simulink model "IMcontrol0"  (Simulink 10.0)
settings: Solver=ode23tb  StartTime=0.0  StopTime=1  MaxStep=1e-4  RelTol=1e-3
undefined symbols (not defined in the file): DiscIntNeverNeededParam
libraries: powerlib x4, simulink x1
settings Model: Creator=80573  LastModifiedBy=Inspiron
settings DataIOCC: SaveFormat=Dataset
settings OptimizationCC: LifeSpan=auto
settings DebuggingCC: UnderspecifiedInitializationDetection=Simplified  MergeDetectMultiDrivingBlocksExec=error  SFUnexpectedBacktrackingDiag=error  SFNoUnconditionalDefaultTransitionDiag=error  SFExecutionAtInitializationDiag=warning
settings HardwareCC: ProdBitPerPointer=64  ProdBitPerSizeT=64  ProdBitPerPtrDiffT=64  ProdLargestAtomicFloat=Float  ProdIntDivRoundTo=Zero  ProdEndianess=LittleEndian  ProdWordSize=64  ProdHWDeviceType=Intel->x86-64 (Windows64)
settings ModelReferenceCC: PropagateSignalLabelsOutOfModel=on
settings CodeAppCC: StateflowObjectComments=off
settings GRTTargetCC: TargetLangStandard=C99 (ISO)  CombineOutputUpdateFcns=on  GRTInterface=off
settings ConfigComp: CovMetricSettings=dwe  CovHtmlReporting=off  CovSaveCumulativeToWorkspaceVar=off  CovSaveSingleToWorkspaceVar=off

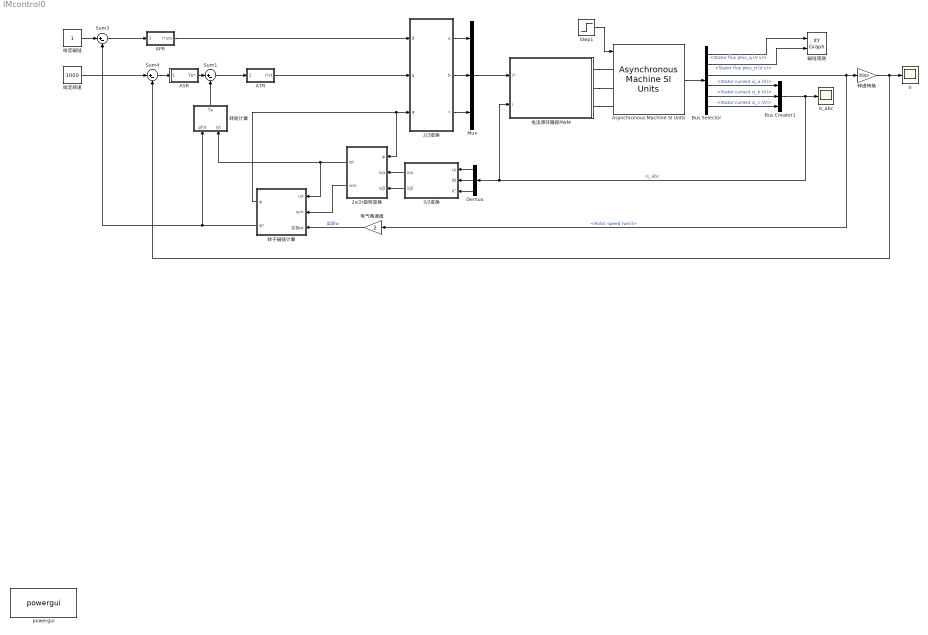
== system IMcontrol0 ==
  2/3变换 : Subsystem
  2s/2r旋转变换 : Subsystem
  3/2变换 : Subsystem
  AFR : Subsystem
  ASR : Subsystem
  ATR : Subsystem
  Asynchronous Machine SI Units : powerlib/Machines/Asynchronous Machine SI Units  RotorType=Squirrel-cage  PresetModel=No  MechanicalLoad=Torque Tm  ShowDetailedParameters=on  ReferenceFrame=Stationary  Units=SI  MeasurementBus=off  NominalParameters=[2200 380 50]  Stator=[0.435 0.002]  Rotor=[0.816 0.002]  Cage1=[0.4155 0.002066]  Cage2=[0.4168 0.0003495]  Lm=0.069  Mechanical=[0.19 0 2]  PolePairs=2  InitialConditions=[1 0 0 0 0 0 0 0]  SimulateSaturation=off  Saturation=[14.03593122, 27.81365428, 53.79336849, 72.68890987, 97.98006896, 148.6815601, 215.7428561, 302.9841135, 428.7778367 ; 230, 322, 414, 460, 506, 552, 598, 644, 690]  LoadFlowParameters=1492000  TsPowergui=0  TsBlock=-1  IterativeModel=Trapezoidal non iterative  IterativeDiscreteModel=Trapezoidal non iterative  Pmec=1.492e+006
      settings: SourceProductName=Simscape Electrical
  Bus Creator1 : BusCreator  Inputs=3
  Bus Selector : BusSelector  OutputSignals=Stator measurements.Stator flux phis_q (V s),Stator measurements.Stator flux phis_d (V s),Mechanical.Rotor speed (wm),Stator measurements.Stator current is_a (A),Stator measurements.Stator current is_b (A),Stator measurements.Stator current is_c (A)
  Demux : Demux  Outputs=3
  Mux : Mux  Inputs=3
  Step1 : Step  Time=0.6  After=55  SampleTime=0
  Sum1 : Sum  Inputs=|+-
  Sum3 : Sum  Inputs=|+-
  Sum4 : Sum  Inputs=|+-
  is_abc : Scope
  n : Scope
  powergui : powerlib/powergui  SimulationMode=Discrete  SampleTime=0.00001  frequency=50  Iterations=50  frequencyindice=50  Pbase=100e6  ErrMax=1e-4  UnitsV=kV  UnitsW=MW  buscounter=0  FunctionMessages=off  echomessages=off  EnableUseOfTLC=off  CurrentSourceSwitches=off  DisableSnubberDevices=off  DisableRonSwitches=off  DisableVfSwitches=off  DisplayEquations=off  AutomaticDiscreteSolvers=off  SolverType=Tustin/Backward Euler (TBE)  Interpol=off  ExternalGateDelay=off  methode=off  Ts=100  x0status=zero  SPID=on  SwTol=0  HookPort=off  NonlinearTolerance=1e-4  nMaxIteration=100  ContinueOnMaxIteration=off  RestoreLinks=warning  ResistiveCurrentMeasurement=off  Frange=[0:2:500]  Ylog=off  Xlog=on  ShowGrid=off  save=off  variable=ZData  structure=0  ZoomFFT=on  StartTime=0.0  cycles=1  DisplayStyle=1  fundamental=60  FreqAxis=off  MaxFrequency=1000  frequencyindicesteady=1  RmsSteady=1  display=off
      settings: SourceProductName=Simscape Electrical
  电气角速度 : Gain  Gain=2
  电流滞环跟踪PWM : Subsystem
  磁链观测 : simulink/Sinks/XY Graph  xmin=-1  xmax=1  ymin=-1  ymax=1  st=-1
  给定磁链 : Constant
  给定转速 : Constant  Value=1000
  转子磁链计算 : Subsystem
  转矩计算 : MATLAB Function  TreatAsAtomicUnit=on
  转速转换 : Gain  Gain=30/pi
  wires:
  Step1/1 -> Asynchronous Machine SI Units/1
  Sum1/1 -> ATR/1(" ")
  Sum3/1 -> AFR/1(" ")
  Sum4/1 -> ASR/1("  ")
  给定磁链/1 -> Sum3/1
  ATR/1(i*st) -> 2/3变换/2(q)
  2/3变换/2(b) -> Mux/2
  2/3变换/3(c) -> Mux/3
  AFR/1(i*sm) -> 2/3变换/1(d)
  2/3变换/1(a) -> Mux/1
  Bus Selector/4 -> Bus Creator1/1  "<Stator current is_a (A)>"
  Bus Selector/6 -> Bus Creator1/3  "<Stator current is_c (A)>"
  Bus Selector/1 -> 磁链观测/1  "<Stator flux phis_q (V s)>"
  Bus Selector/2 -> 磁链观测/2  "<Stator flux phis_d (V s)>"
  Bus Selector/5 -> Bus Creator1/2  "<Stator current is_b (A)>"
  Bus Selector/3 -> 电气角速度/1, 转速转换/1  "<Rotor speed (wm)>"
  Bus Creator1/1 -> 电流滞环跟踪PWM/2(i), Demux/1, is_abc/1  "is_abc"
  Asynchronous Machine SI Units/1 -> Bus Selector/1
  Mux/1 -> 电流滞环跟踪PWM/1(i*)
  ASR/1(Te*) -> Sum1/1
  转矩计算/1(Te) -> Sum1/2
  Demux/1 -> 3/2变换/1(iA)
  Demux/2 -> 3/2变换/2(iB)
  Demux/3 -> 3/2变换/3(iC)
  2s/2r旋转变换/1(ist) -> 转矩计算/2(ist), 转子磁链计算/1(ist)
  3/2变换/1(isα) -> 2s/2r旋转变换/2(isα)
  3/2变换/2(isβ) -> 2s/2r旋转变换/3(isβ)
  给定转速/1 -> Sum4/1
  转速转换/1 -> Sum4/2, n/1
  转子磁链计算/2(ψr) -> Sum3/2, 转矩计算/1(phir)
  转子磁链计算/1(φ) -> 2s/2r旋转变换/1(φ), 2/3变换/3(φ)
  电气角速度/1 -> 转子磁链计算/3(实际w)  "实际w"
  2s/2r旋转变换/2(ism) -> 转子磁链计算/2(ism)
  connections:
  电流滞环跟踪PWM/RConn1 -- Asynchronous Machine SI Units/LConn1
  电流滞环跟踪PWM/RConn2 -- Asynchronous Machine SI Units/LConn2
  电流滞环跟踪PWM/RConn3 -- Asynchronous Machine SI Units/LConn3

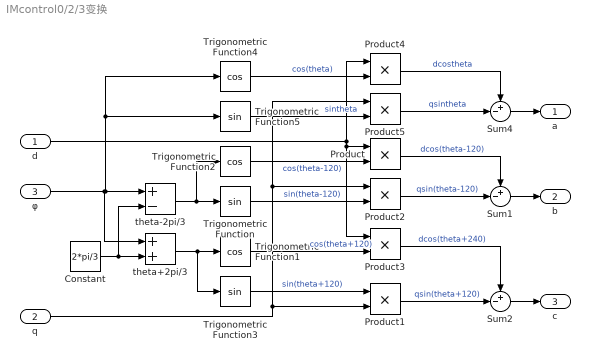
== system IMcontrol0/2/3变换 ==
  d : Inport
  q : Inport  Port=2
  φ : Inport  Port=3
  Constant : Constant  Value=2*pi/3
  Product{,1..5} (6 alike) : Product
  Sum1 : Sum  Inputs=+-|
  Sum2 : Sum  Inputs=+-|
  Sum4 : Sum  Inputs=+-|
  Trigonometric Function : Trigonometry
  Trigonometric Function1 : Trigonometry  Operator=cos
  Trigonometric Function2 : Trigonometry  Operator=cos
  Trigonometric Function3 : Trigonometry
  Trigonometric Function4 : Trigonometry  Operator=cos
  Trigonometric Function5 : Trigonometry
  theta+2pi/3 : Sum
  theta-2pi/3 : Sum  Inputs=+-
  a : Outport  VectorParamsAs1DForOutWhenUnconnected=off
  b : Outport  Port=2  VectorParamsAs1DForOutWhenUnconnected=off
  c : Outport  Port=3  VectorParamsAs1DForOutWhenUnconnected=off
  wires:
  Trigonometric Function5/1 -> Product5/2  "sintheta"
  Product/1 -> Sum1/1  "dcos(theta-120)"
  Trigonometric Function1/1 -> Product3/2  "cos(theta+120)"
  Product3/1 -> Sum2/1  "dcos(theta+240)"
  d/1 -> Product/1, Product3/1, Product4/1
  Constant/1 -> theta+2pi/3/2, theta-2pi/3/2
  φ/1 -> Trigonometric Function4/1, Trigonometric Function5/1, theta-2pi/3/1, theta+2pi/3/1
  theta+2pi/3/1 -> Trigonometric Function3/1, Trigonometric Function1/1
  q/1 -> Product5/1, Product2/1, Product1/2
  Trigonometric Function/1 -> Product2/2  "sin(theta-120)"
  Product4/1 -> Sum4/1  "dcostheta"
  Product5/1 -> Sum4/2  "qsintheta"
  theta-2pi/3/1 -> Trigonometric Function2/1, Trigonometric Function/1
  Product1/1 -> Sum2/2  "qsin(theta+120)"
  Trigonometric Function2/1 -> Product/2  "cos(theta-120)"
  Sum4/1 -> a/1
  Sum1/1 -> b/1
  Trigonometric Function4/1 -> Product4/2  "cos(theta)"
  Trigonometric Function3/1 -> Product1/1  "sin(theta+120)"
  Product2/1 -> Sum1/2  "qsin(theta-120)"
  Sum2/1 -> c/1

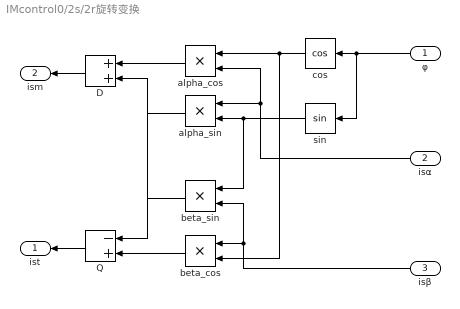
== system IMcontrol0/2s/2r旋转变换 ==
  φ : Inport
  isα : Inport  Port=2
  isβ : Inport  Port=3
  D : Sum
  Q : Sum  Inputs=-+
  alpha_cos : Product
  alpha_sin : Product
  beta_cos : Product
  beta_sin : Product
  cos : Trigonometry  Operator=cos
  sin : Trigonometry
  ist : Outport
  ism : Outport  Port=2
  wires:
  cos/1 -> beta_cos/2, alpha_cos/1
  beta_cos/1 -> Q/2
  sin/1 -> beta_sin/1, alpha_sin/2
  isα/1 -> alpha_cos/2, alpha_sin/1
  alpha_sin/1 -> Q/1
  beta_sin/1 -> D/2
  isβ/1 -> beta_sin/2, beta_cos/1
  φ/1 -> sin/1, cos/1
  D/1 -> ism/1
  alpha_cos/1 -> D/1
  Q/1 -> ist/1

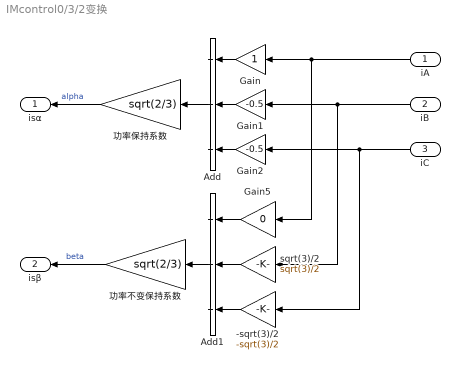
== system IMcontrol0/3/2变换 ==
  iA : Inport
  iB : Inport  Port=2
  iC : Inport  Port=3
  -sqrt(3)/2 : Gain  Gain=-sqrt(3)/2
  Add : Sum  Inputs=3
  Add1 : Sum  Inputs=3
  Gain : Gain
  Gain1 : Gain  Gain=-0.5
  Gain2 : Gain  Gain=-0.5
  Gain5 : Gain  Gain=0
  sqrt(3)/2 : Gain  Gain=sqrt(3)/2
  功率不变保持系数 : Gain  Gain=sqrt(2/3)
  功率保持系数 : Gain  Gain=sqrt(2/3)
  isα : Outport
  isβ : Outport  Port=2
  wires:
  sqrt(3)/2/1 -> Add1/2
  Gain/1 -> Add/1
  -sqrt(3)/2/1 -> Add1/3
  iB/1 -> sqrt(3)/2/1, Gain1/1
  Add/1 -> 功率保持系数/1
  Gain1/1 -> Add/2
  Gain5/1 -> Add1/1
  iA/1 -> Gain5/1, Gain/1
  Gain2/1 -> Add/3
  iC/1 -> -sqrt(3)/2/1, Gain2/1
  Add1/1 -> 功率不变保持系数/1
  功率不变保持系数/1 -> isβ/1  "beta"
  功率保持系数/1 -> isα/1  "alpha"

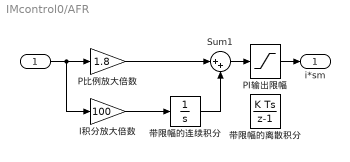
== system IMcontrol0/AFR ==
  " " : Inport
  I积分放大倍数 : Gain  Gain=100
  PI输出限幅 : Saturate  UpperLimit=13  LowerLimit=-13
  P比例放大倍数 : Gain  Gain=1.8
  Sum1 : Sum  Inputs=|++
  带限幅的离散积分 : DiscreteIntegrator  SampleTime=2e-5  ICPrevOutput=DiscIntNeverNeededParam  ICPrevScaledInput=DiscIntNeverNeededParam
  带限幅的连续积分 : Integrator  LimitOutput=on  UpperSaturationLimit=15  LowerSaturationLimit=-15
  i*sm : Outport  VectorParamsAs1DForOutWhenUnconnected=off
  wires:
  Sum1/1 -> PI输出限幅/1
  PI输出限幅/1 -> i*sm/1
  I积分放大倍数/1 -> 带限幅的连续积分/1
  P比例放大倍数/1 -> Sum1/1
  带限幅的连续积分/1 -> Sum1/2
  " "/1 -> I积分放大倍数/1, P比例放大倍数/1

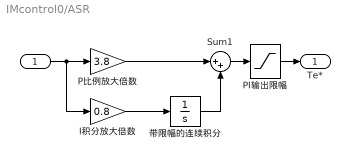
== system IMcontrol0/ASR ==
  "  " : Inport
  I积分放大倍数 : Gain  Gain=0.8
  PI输出限幅 : Saturate  UpperLimit=75  LowerLimit=-75
  P比例放大倍数 : Gain  Gain=3.8
  Sum1 : Sum  Inputs=|++
  带限幅的连续积分 : Integrator  LimitOutput=on  UpperSaturationLimit=80  LowerSaturationLimit=-80
  Te* : Outport  VectorParamsAs1DForOutWhenUnconnected=off
  wires:
  Sum1/1 -> PI输出限幅/1
  PI输出限幅/1 -> Te*/1
  P比例放大倍数/1 -> Sum1/1
  I积分放大倍数/1 -> 带限幅的连续积分/1
  带限幅的连续积分/1 -> Sum1/2
  "  "/1 -> I积分放大倍数/1, P比例放大倍数/1

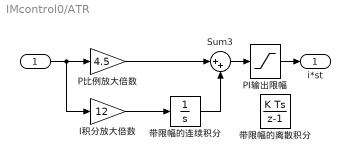
== system IMcontrol0/ATR ==
  " " : Inport
  I积分放大倍数 : Gain  Gain=12
  PI输出限幅 : Saturate  UpperLimit=60  LowerLimit=-60
  P比例放大倍数 : Gain  Gain=4.5
  Sum3 : Sum  Inputs=|++
  带限幅的离散积分 : DiscreteIntegrator  SampleTime=2e-5  ICPrevOutput=DiscIntNeverNeededParam  ICPrevScaledInput=DiscIntNeverNeededParam
  带限幅的连续积分 : Integrator  LimitOutput=on  UpperSaturationLimit=65  LowerSaturationLimit=-65
  i*st : Outport  VectorParamsAs1DForOutWhenUnconnected=off
  wires:
  Sum3/1 -> PI输出限幅/1
  P比例放大倍数/1 -> Sum3/1
  " "/1 -> I积分放大倍数/1, P比例放大倍数/1
  PI输出限幅/1 -> i*st/1
  带限幅的连续积分/1 -> Sum3/2
  I积分放大倍数/1 -> 带限幅的连续积分/1

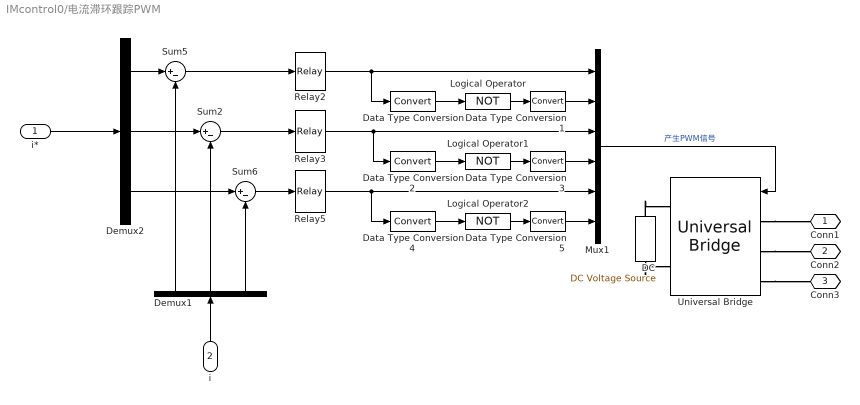
== system IMcontrol0/电流滞环跟踪PWM ==
  i* : Inport
  i : Inport  Port=2
  DC : powerlib/Electrical Sources/DC Voltage Source  Amplitude=510  Measurements=None
      settings: SourceProductName=Simscape Electrical
  Data Type Conversion{,1..5} (6 alike) : DataTypeConversion
  Demux1 : Demux  Outputs=3
  Demux2 : Demux  Outputs=3
  Logical Operator : Logic  Operator=NOT  Inputs=1  AllPortsSameDT=off
  Logical Operator1 : Logic  Operator=NOT  Inputs=1  AllPortsSameDT=off
  Logical Operator2 : Logic  Operator=NOT  Inputs=1  AllPortsSameDT=off
  Mux1 : Mux  Inputs=6
  Relay2 : Relay  OnSwitchValue=0.2  OffSwitchValue=-0.2  ZeroCross=off
  Relay3 : Relay  OnSwitchValue=0.2  OffSwitchValue=-0.2  ZeroCross=off
  Relay5 : Relay  OnSwitchValue=0.2  OffSwitchValue=-0.2  ZeroCross=off
  Sum2 : Sum  Inputs=|+-
  Sum5 : Sum  Inputs=|+-
  Sum6 : Sum  Inputs=|+-
  Universal Bridge : powerlib/Power Electronics/Universal Bridge  Arms=3  SnubberResistance=1e5  SnubberCapacitance=inf  Device=IGBT / Diodes  Ron=1e-3  Lon=0  ForwardVoltages="[  0  0  ]"  ForwardVoltage=0  GTOparameters=[ 10e-6 , 20e-6 ]  IGBTparameters=[ 1e-6 , 2e-6 ]  Measurements=None  Measurements_2=None  converterType=Rectifier
      settings: SourceProductName=Simscape Electrical
  Conn1 : PMIOPort  Side=Right
  Conn2 : PMIOPort  Port=2  Side=Right
  Conn3 : PMIOPort  Port=3  Side=Right
  wires:
  Sum6/1 -> Relay5/1
  Data Type Conversion1/1 -> Mux1/2
  Sum5/1 -> Relay2/1
  Relay5/1 -> Data Type Conversion4/1, Mux1/5
  Data Type Conversion3/1 -> Mux1/4
  Relay2/1 -> Data Type Conversion/1, Mux1/1
  Relay3/1 -> Data Type Conversion2/1, Mux1/3
  Mux1/1 -> Universal Bridge/1  "产生PWM信号"
  Demux1/3 -> Sum6/2
  i/1 -> Demux1/1
  Demux2/1 -> Sum5/1
  Logical Operator2/1 -> Data Type Conversion5/1
  Data Type Conversion/1 -> Logical Operator/1
  i*/1 -> Demux2/1
  Logical Operator/1 -> Data Type Conversion1/1
  Demux1/2 -> Sum2/2
  Data Type Conversion5/1 -> Mux1/6
  Data Type Conversion2/1 -> Logical Operator1/1
  Demux1/1 -> Sum5/2
  Demux2/3 -> Sum6/1
  Demux2/2 -> Sum2/1
  Data Type Conversion4/1 -> Logical Operator2/1
  Sum2/1 -> Relay3/1
  Logical Operator1/1 -> Data Type Conversion3/1
  connections:
  DC/LConn1 -- Universal Bridge/RConn2
  DC/RConn1 -- Universal Bridge/RConn1
  Universal Bridge/LConn1 -- Conn1/RConn1
  Universal Bridge/LConn2 -- Conn2/RConn1
  Universal Bridge/LConn3 -- Conn3/RConn1

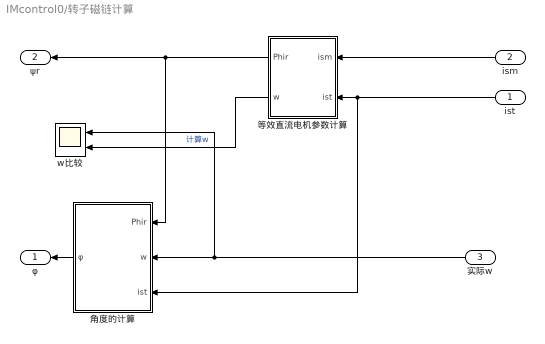
== system IMcontrol0/转子磁链计算 ==
  ist : Inport
  ism : Inport  Port=2
  实际w : Inport  Port=3
  w比较 : Scope  NumInputPorts=2
  等效直流电机参数计算 : Subsystem
  角度的计算 : Subsystem
  φ : Outport
  ψr : Outport  Port=2
  wires:
  等效直流电机参数计算/1(Phir) -> ψr/1, 角度的计算/1(Phir)
  实际w/1 -> w比较/1, 角度的计算/2(w)
  ist/1 -> 角度的计算/3(ist), 等效直流电机参数计算/2(ist)
  等效直流电机参数计算/2(w) -> w比较/2  "计算w"
  角度的计算/1(φ) -> φ/1
  ism/1 -> 等效直流电机参数计算/1(ism)

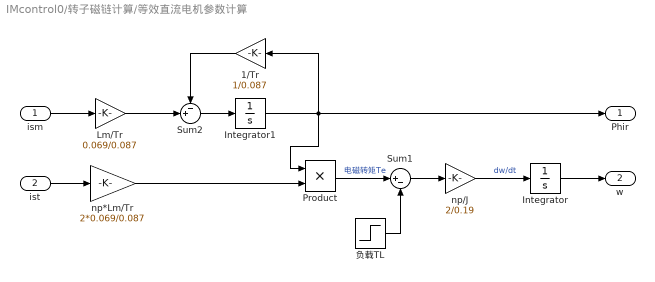
== system IMcontrol0/转子磁链计算/等效直流电机参数计算 ==
  ism : Inport
  ist : Inport  Port=2
  1/Tr : Gain  Gain=1/0.087
  Integrator : Integrator
  Integrator1 : Integrator  InitialCondition=1e-5
  Lm/Tr : Gain  Gain=0.069/0.087
  Product : Product
  Sum1 : Sum  Inputs=|+-
  Sum2 : Sum  Inputs=-+|
  np*Lm/Tr : Gain  Gain=2*0.069/0.087
  np/J : Gain  Gain=2/0.19
  负载TL : Step  Time=0.6  After=55  SampleTime=0
  Phir : Outport  VectorParamsAs1DForOutWhenUnconnected=off
  w : Outport  Port=2  VectorParamsAs1DForOutWhenUnconnected=off
  wires:
  Sum2/1 -> Integrator1/1
  Integrator1/1 -> Phir/1, Product/1, 1/Tr/1
  Sum1/1 -> np/J/1
  np*Lm/Tr/1 -> Product/2
  ism/1 -> Lm/Tr/1
  Lm/Tr/1 -> Sum2/2
  ist/1 -> np*Lm/Tr/1
  Integrator/1 -> w/1
  负载TL/1 -> Sum1/2
  np/J/1 -> Integrator/1  "dw/dt"
  Product/1 -> Sum1/1  "电磁转矩Te"
  1/Tr/1 -> Sum2/1

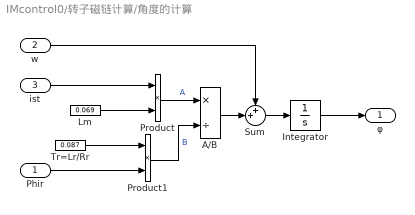
== system IMcontrol0/转子磁链计算/角度的计算 ==
  Phir : Inport
  w : Inport  Port=2
  ist : Inport  Port=3
  A/B : Product  Inputs=*/
  Integrator : Integrator
  Lm : Constant  Value=0.069
  Product : Product
  Product1 : Product
  Sum : Sum  Inputs=++|
  Tr=Lr/Rr : Constant  Value=0.087
  φ : Outport  VectorParamsAs1DForOutWhenUnconnected=off
  wires:
  ist/1 -> Product/1
  w/1 -> Sum/1
  Product/1 -> A/B/1  "A"
  Sum/1 -> Integrator/1
  Integrator/1 -> φ/1
  Product1/1 -> A/B/2  "B"
  Lm/1 -> Product/2
  A/B/1 -> Sum/2
  Phir/1 -> Product1/2
  Tr=Lr/Rr/1 -> Product1/1

== matlab function 转矩计算 ==
  data: phir input double; Te output double; ist input double
function Te  = fcn(phir,ist)
Te=2*0.069*phir*ist/0.071
%Te=np（磁极对数）*Lm*phir*ist/Lr
